simulink model "obsv"  (R2021a)
settings: Solver=VariableStepAuto  StartTime=0.0  StopTime=10.0  RelTol=1e-3
undefined symbols (not defined in the file or in its folder): A, Ao, B, Bo, C, Co, D, Do, K
settings Model: Creator=itama  LastModifiedBy=itama

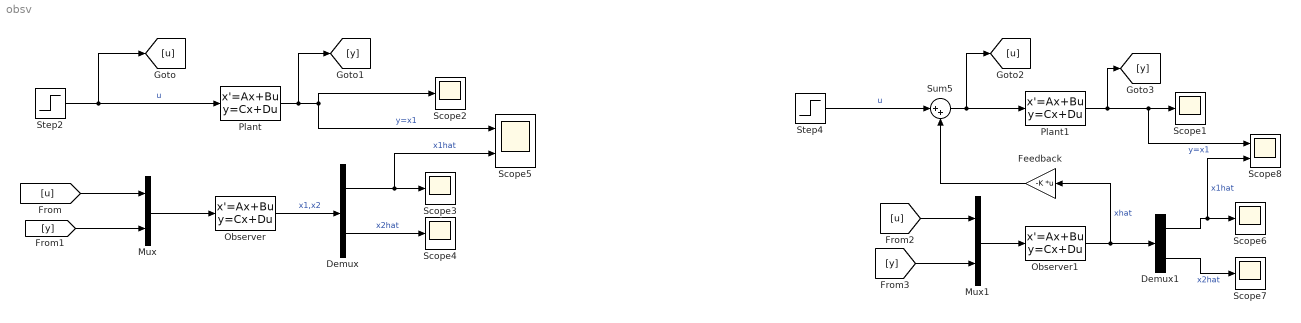
== system obsv ==
  Demux : Demux  Outputs=2
  Demux1 : Demux  Outputs=2
  Feedback : Gain  Gain=-K  Multiplication=Matrix(K*u)
  Mux : Mux  Inputs=2
  Mux1 : Mux  Inputs=2
  Observer : StateSpace  A=Ao  B=Bo  C=Co  D=Do  InitialCondition=[0;0]
  Observer1 : StateSpace  A=Ao  B=Bo  C=Co  D=Do  InitialCondition=[0;0]
  Plant : StateSpace  A=A  B=B  C=C  D=D  InitialCondition=[0;0]
  Plant1 : StateSpace  A=A  B=B  C=C  D=D  InitialCondition=[0;0]
  Scope{1..4,6..7} (6 alike) : Scope
  Scope5 : Scope  NumInputPorts=2
  Scope8 : Scope  NumInputPorts=2
  Step2 : Step  SampleTime=0
  Step4 : Step  Time=0  SampleTime=0
  Sum5 : Sum  Inputs=|++
  wires:
  Observer/1 -> Demux/1  "x1,x2"
  [u] -> Mux/1
  Demux/2 -> Scope4/1  "x2hat"
  Mux/1 -> Observer/1
  Step2/1 -> [u], Plant/1  "u"
  Plant/1 -> [y], Scope5/1, Scope2/1  "y=x1"
  Demux/1 -> Scope5/2, Scope3/1  "x1hat"
  [y] -> Mux/2
  Feedback/1 -> Sum5/2
  [y] -> Mux1/2
  Sum5/1 -> [u], Plant1/1
  Demux1/1 -> Scope8/2, Scope6/1  "x1hat"
  Demux1/2 -> Scope7/1  "x2hat"
  [u] -> Mux1/1
  Plant1/1 -> [y], Scope8/1, Scope1/1  "y=x1"
  Step4/1 -> Sum5/1  "u"
  Observer1/1 -> Feedback/1, Demux1/1  "xhat"
  Mux1/1 -> Observer1/1
